simulink model "PEnergyMeter"  (R2024b)
settings: Solver=FixedStepAuto  StartTime=0.0  StopTime=10.0  RelTol=1e-3  EnableMultiTasking=on
undefined symbols (not defined in the file): PRulesLimit
settings Model: DataDictionary=Master_Dictionary.sldd  EnableAccessToBaseWorkspace=off  Creator=ella  LastModifiedBy=Will
settings OptimizationCC: DefaultParameterBehavior=Inlined  EnhancedBackFolding=on  PassReuseOutputArgsAs=Individual arguments  ZeroExternalMemoryAtStartup=off  ZeroInternalMemoryAtStartup=off  MaxStackSize=8192  OptimizeBlockOrder=speed  DifferentSizesBufferReuse=on  OptimizationCustomize=off  EfficientTunableParamExpr=on
settings DebuggingCC: ParameterTunabilityLossMsg=error
settings HardwareCC: ProdBitPerPointer=32  ProdBitPerSizeT=32  ProdBitPerPtrDiffT=32  ProdLargestAtomicInteger=Long  ProdLargestAtomicFloat=Double  ProdWordSize=32  ProdLongLongMode=on  ProdHWDeviceType=ARM Compatible->ARM Cortex-M
settings SFSimCC: MATLABDynamicMemAlloc=off
settings RTWCC: Description=Embedded Coder  SystemTargetFile=ert.tlc  HardwareBoard=STM32H7xx Based (Single-core)  TemplateMakefile=ert_default_tmf  Toolchain=GNU Tools for ARM Embedded Processors
settings CodeAppCC: ForceParamTrailComments=on  IgnoreCustomStorageClasses=off  OperatorAnnotations=on  SimulinkDataObjDesc=on  SFDataObjDesc=on  InsertBlockDesc=on
settings ERTTargetCC: TargetLangStandard=C99 (ISO)  CodeReplacementLibrary=ARM Cortex-M  ExtModeTransport=3  ExtModeStaticAlloc=on  ExtModeStaticAllocSize=2048  ExtModeMexFile=ext_xcp  ExtModeIntrfLevel=Level2 - Open

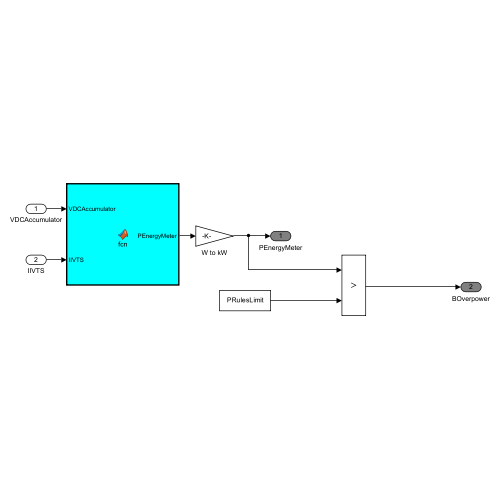
[thumbnail: Simulink's stored preview of the top-level diagram]
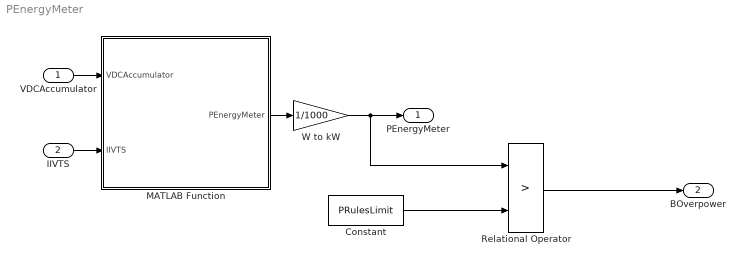
== system PEnergyMeter ==
  "VDCAccumulator " : Inport  OutDataTypeStr=double
  "IIVTS " : Inport  Port=2  OutDataTypeStr=double
  Constant : Constant  Value=PRulesLimit  SampleTime=-1
  MATLAB Function : MATLAB Function  TreatAsAtomicUnit=on
      settings: MinAlgLoopOccurrences=on
  Relational Operator : RelationalOperator  Operator=>  OutDataTypeStr=boolean  RndMeth=Simplest  InputSameDT=off
  W to kW : Gain  Gain=1/1000
  "PEnergyMeter " : Outport  OutDataTypeStr=double  VectorParamsAs1DForOutWhenUnconnected=off
  "BOverpower " : Outport  Port=2  OutDataTypeStr=boolean  VectorParamsAs1DForOutWhenUnconnected=off
  wires:
  "VDCAccumulator "/1 -> MATLAB Function/1(VDCAccumulator)
  "IIVTS "/1 -> MATLAB Function/2(IIVTS)
  MATLAB Function/1(PEnergyMeter) -> W to kW/1
  W to kW/1 -> Relational Operator/1, "PEnergyMeter "/1
  Constant/1 -> Relational Operator/2
  Relational Operator/1 -> "BOverpower "/1

== matlab function PEnergyMeter/MATLAB Function ==
  data: VDCAccumulator input; PEnergyMeter output; IIVTS input
function PEnergyMeter = fcn(VDCAccumulator, IIVTS)
% rolling avg of 500ms (window)
% multiplies VIn*IIn average over 500ms
% frequency assumption 1kHz? Ts = 0.001s 

%run
persistent buffer N 
if isempty(N)
%Ts =  0.001;        % sample time (s)
%window = 0.5; % 500ms window
%N = round(window/Ts); % number of samples in window
N = 500;
buffer = zeros(1,500);  % initialise buffer
end 
 
% calculate instantaneous power
P_inst = VDCAccumulator * IIVTS;
 
% update rolling buffer 
buffer = [buffer(2:end), P_inst];
 
%compute mean power over last 500ms 
PEnergyMeter = mean(buffer); 
end
